simulink model "lab3mots"  (R2022a)
settings: Solver=VariableStepAuto  StartTime=0.0  StopTime=20  MaxStep=0.00001  MinStep=0.000001  RelTol=1e-3
model workspace (MAT data in the model file):
  J = 0.000108
  K = 100
  kb = 0.0136
  km = 23.32
undefined symbols (not defined in the file or in its folder): k, q_1, q_2, T, y_0
settings Model: Creator=Дмитрий  LastModifiedBy=Дмитрий

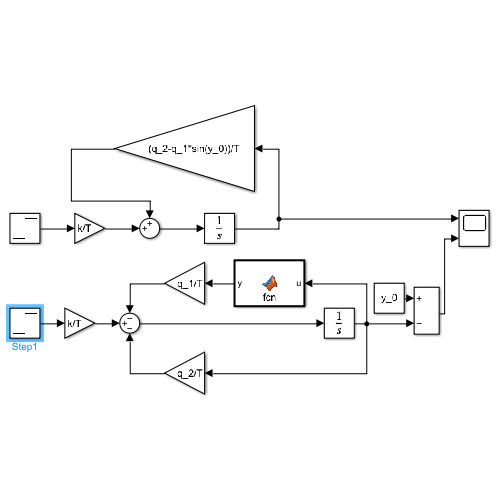
[thumbnail: Simulink's stored preview of the top-level diagram]
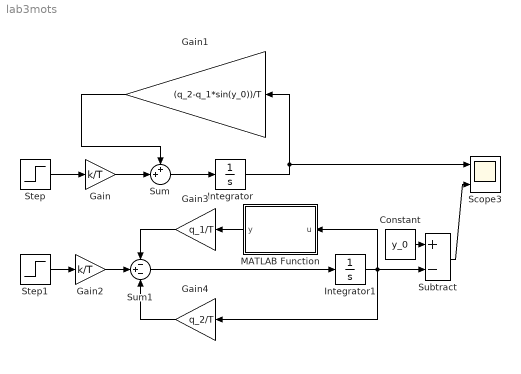
== system lab3mots ==
  Constant : Constant  Value=y_0
  Gain : Gain  Gain=k/T
  Gain1 : Gain  Gain=(q_2-q_1*sin(y_0))/T
  Gain2 : Gain  Gain=k/T
  Gain3 : Gain  Gain=q_1/T
  Gain4 : Gain  Gain=q_2/T
  Integrator : Integrator
  Integrator1 : Integrator  InitialCondition=y_0
  MATLAB Function : MATLAB Function  TreatAsAtomicUnit=on
  Scope3 : Scope  NumInputPorts=2
  Step : Step  Before=1  SampleTime=0
  Step1 : Step  Time=1+1.22  Before=1  SampleTime=0
  Subtract : Sum  Inputs=+-
  Sum : Sum  Inputs=++|
  Sum1 : Sum  Inputs=-+-
  wires:
  Step/1 -> Gain/1
  Gain/1 -> Sum/2
  Sum/1 -> Integrator/1
  Gain1/1 -> Sum/1
  Integrator/1 -> Gain1/1, Scope3/1
  Step1/1 -> Gain2/1
  Gain2/1 -> Sum1/2
  Gain3/1 -> Sum1/1
  Gain4/1 -> Sum1/3
  Sum1/1 -> Integrator1/1
  MATLAB Function/1(y) -> Gain3/1
  Subtract/1 -> Scope3/2
  Integrator1/1 -> Gain4/1, MATLAB Function/1(u), Subtract/2
  Constant/1 -> Subtract/1

== matlab function lab3mots/MATLAB Function ==
  data: u input; y output
function y = fcn(u)

y = cos(u);
